simulink model "AMtiaozhi"  (R2018a)
settings: Solver=VariableStepAuto  StartTime=0.0  StopTime=50.0  RelTol=1e-3
libraries: dsparch4 x1
settings Model: Creator=mengmeng  LastModifiedBy=mengmeng

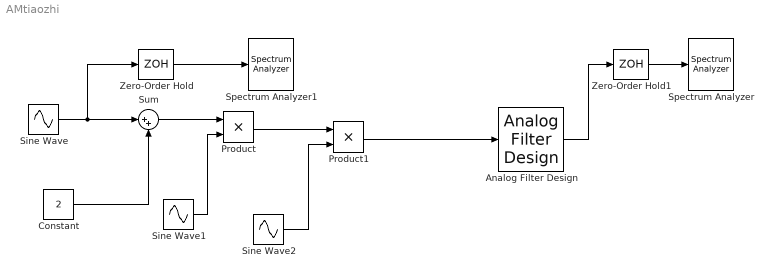
== system AMtiaozhi ==
  Analog Filter Design : dsparch4/Analog Filter Design  method=Butterworth  filttype=Lowpass  N=8  Wlo=500  Whi=80  Rp=2  Rs=40
  Constant : Constant  Value=2
  Product : Product
  Product1 : Product
  Sine Wave : Sin  Frequency=500  SampleTime=0
  Sine Wave1 : Sin  Frequency=6000  SampleTime=0
  Sine Wave2 : Sin  Frequency=6000  SampleTime=0
  Spectrum Analyzer : SpectrumAnalyzer
  Spectrum Analyzer1 : SpectrumAnalyzer
  Sum : Sum  Inputs=|++
  Zero-Order Hold : ZeroOrderHold  SampleTime=0.01
  Zero-Order Hold1 : ZeroOrderHold  SampleTime=0.01
  wires:
  Sine Wave/1 -> Zero-Order Hold/1, Sum/1
  Constant/1 -> Sum/2
  Sum/1 -> Product/1
  Sine Wave1/1 -> Product/2
  Product/1 -> Product1/1
  Sine Wave2/1 -> Product1/2
  Product1/1 -> Analog Filter Design/1
  Zero-Order Hold1/1 -> Spectrum Analyzer/1
  Zero-Order Hold/1 -> Spectrum Analyzer1/1
  Analog Filter Design/1 -> Zero-Order Hold1/1
